simulink model "InvLamp"  (Simulink 4.00)
settings: Solver=ode45  SolverMode=SingleTasking  StartTime=0.0  StopTime=10.0  RelTol=1e-3  AbsTol=1e-6
settings Model: LastModifiedBy=abbas  LimitDataPoints=off  BlockReductionOpt=off

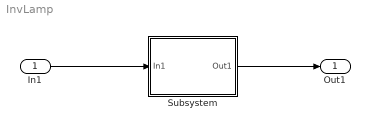
== system InvLamp ==
  In1 : Inport  Port=1
  Subsystem : Subsystem
      settings: RTWFcnNameOpts=Auto  RTWFileNameOpts=Auto
  Out1 : Outport  Port=1
  wires:
  In1/1 -> Subsystem/1(In1)
  Subsystem/1(Out1) -> Out1/1

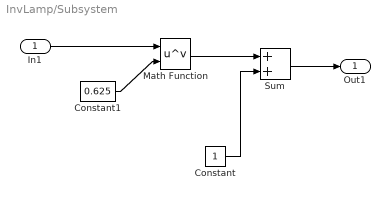
== system InvLamp/Subsystem ==
  In1 : Inport  Port=1
  Constant : Constant  Value=1
  Constant1 : Constant  Value=0.625
  Math Function : Math  Operator=pow  OutputSignalType=auto
  Sum : Sum  Inputs=++  SaturateOnIntegerOverflow=on
  Out1 : Outport  Port=1
  wires:
  Constant1/1 -> Math Function/2
  Sum/1 -> Out1/1
  Constant/1 -> Sum/2
  In1/1 -> Math Function/1
  Math Function/1 -> Sum/1
